simulink model "gm_fiter_model"  (R2021a)
settings: Solver=VariableStepAuto  StartTime=0.0  StopTime=10.0  RelTol=1e-3
libraries: hdlsllib x3
settings Model: Creator=MGMA  LastModifiedBy=MGMA
settings OptimizationCC: BlockReduction=off  ConditionallyExecuteInputs=off
settings DebuggingCC: InheritedTsInSrcMsg=none

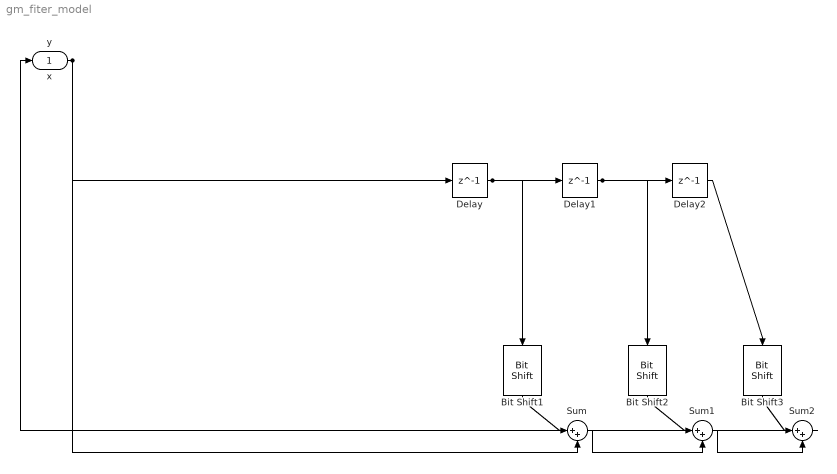
== system gm_fiter_model ==
  x : Inport  OutDataTypeStr=uint8  PortDimensions=1  SampleTime=0.2
  Bit Shift1 : hdlsllib/Logic and Bit Operations/Bit Shift  mode=Shift Right Logical  N=1
  Bit Shift2 : hdlsllib/Logic and Bit Operations/Bit Shift  mode=Shift Right Logical  N=2
  Bit Shift3 : hdlsllib/Logic and Bit Operations/Bit Shift  mode=Shift Right Logical  N=3
  Delay : Delay  DelayLength=1  InitialCondition=0
  Delay1 : Delay  DelayLength=1  InitialCondition=0
  Delay2 : Delay  DelayLength=1  InitialCondition=0
  Sum : Sum  Inputs=|++
  Sum1 : Sum  Inputs=|++
  Sum2 : Sum  Inputs=|++
  y : Outport  OutDataTypeStr=uint8  SampleTime=0.2
  wires:
  x/1 -> Sum/2, Delay/1
  Bit Shift1/1 -> Sum/1
  Bit Shift2/1 -> Sum1/1
  Bit Shift3/1 -> Sum2/1
  Delay/1 -> Bit Shift1/1, Delay1/1
  Delay1/1 -> Bit Shift2/1, Delay2/1
  Delay2/1 -> Bit Shift3/1
  Sum/1 -> Sum1/2
  Sum1/1 -> Sum2/2
  Sum2/1 -> y/1
